simulink model "unpack"  (R2018b)
settings: Solver=VariableStepAuto  StartTime=0.0  StopTime=10.0  RelTol=1e-3
(part 1 of 2)
settings Model: Creator=82358  LastModifiedBy=82358

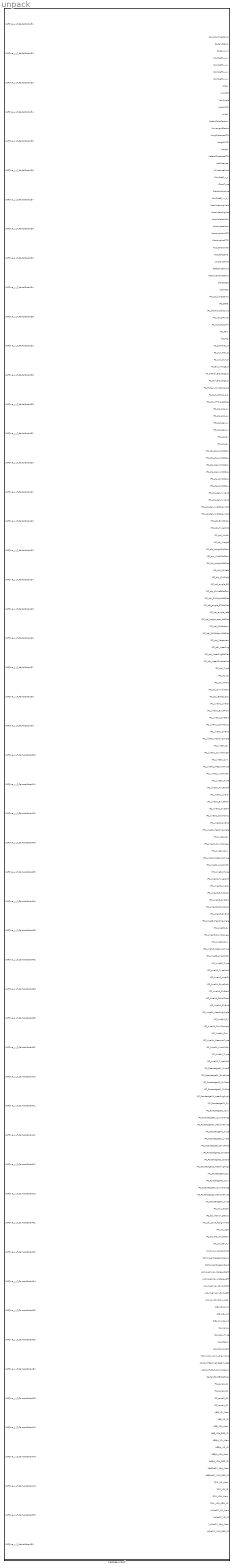
== system unpack ==
  message_unpack : MATLAB Function  TreatAsAtomicUnit=on
